simulink model "Feuchtesimulation_G21_EU6AGA_rueckgabewerte"  (R2021b)
settings: Solver=FixedStepAuto  StartTime=start_time  StopTime=stop_time  FixedStep=ts  RelTol=1e-3
undefined symbols (not defined in the file or in its folder): A_Kat0, A_Kat1, A_Kat2, A_Kat3, A_Mantel_Kat0, A_Mantel_Kat1, A_Mantel_Kat2, A_Mantel_Kat3, Air_N2, Air_O2, beladungskennfeld, C_mw, CO2_mw, FeuchteAnsaugluft_rel, FeuchtegradAnsaugluft, Fuel_C, Fuel_H, H2O_mw, H_mw, Kat0_Anzahl_Zonen, Kat1_Anzahl_Zonen, Kat2_Anzahl_Zonen, Kat3_Anzahl_Zonen, l_Kat0, l_Kat1, l_Kat2, l_Kat3, m_Canning_Kat0, m_Canning_Kat1, m_Canning_Kat2, m_Canning_Kat3, m_h2o_kat0_ads, m_h2o_kat0_kond, m_h2o_kat1_ads, m_h2o_kat1_kond, m_h2o_kat2_ads, m_h2o_kat2_kond, m_h2o_kat3_ads, m_h2o_kat3_kond, m_Isolierung_Kat0, m_Isolierung_Kat1, m_Isolierung_Kat2, m_Isolierung_Kat3, m_zeolith_kat0_zone, m_zeolith_kat1_zone, m_zeolith_kat2_zone, m_zeolith_kat3_zone, m_zKat0, m_zKat1, m_zKat2, m_zKat3, Mat_Kat0, Mat_Kat1, Mat_Kat2, Mat_Kat3, N2_mw, O2_mw, p_dsat, Rohr0, Rohr1 ... (+20)
libraries: Feuchtesimulation_Lib x69
(part 2 of 3)

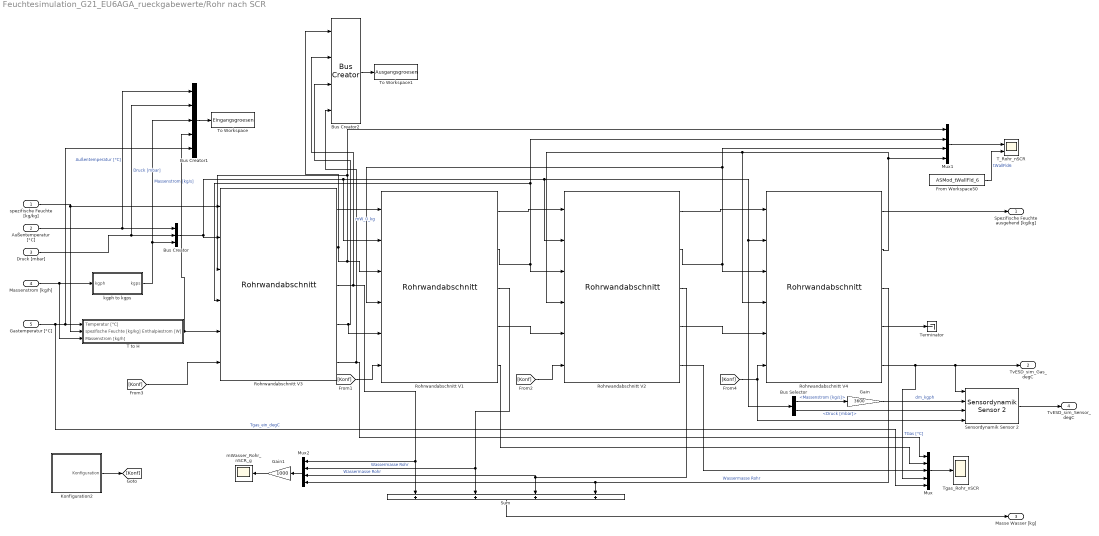
== system Feuchtesimulation_G21_EU6AGA_rueckgabewerte/Rohr nach SCR ==
  spezifische Feuchte [kg/kg] : Inport
  Außentemperatur [°C] : Inport  Port=2
  Druck [mbar] : Inport  Port=3
  Massenstrom [kg/h] : Inport  Port=4
  Gastemperatur [°C] : Inport  Port=5
  Bus Creator : BusCreator  Inputs=3
  Bus Creator1 : BusCreator  Inputs=5
  Bus Creator2 : BusCreator  Inputs=4
  Bus Selector : BusSelector  OutputSignals=Massenstrom [kg/s],Druck [mbar]
  From Workspace50 : FromWorkspace  VariableName=ASMod_tWallFld_6  OutputAfterFinalValue=Holding final value
  Gain : Gain  Gain=3600
  Gain1 : Gain  Gain=1000
  Konfiguration2 : Subsystem
  Mux : Mux  Inputs=5
  Mux1 : Mux
  Mux2 : Mux
  Rohrwandabschnitt V{1..4} (4 alike) : Feuchtesimulation_Lib/Rohrwandabschnitt  SystemSampleTime=-1  VariantActivationTime=update diagram  Latency=0  AutoFrameSizeCalculation=off
  Sensordynamik Sensor 2 : Feuchtesimulation_Lib/Sensordynamik Sensor 2  SystemSampleTime=-1  VariantActivationTime=update diagram  Latency=0  AutoFrameSizeCalculation=off
  Sum : Sum  Inputs=++++
  T to H : Subsystem
  T_Rohr_nSCR : Scope  NumInputPorts=2
  Terminator : Terminator
  Tgas_Rohr_nSCR : Scope
  To Workspace : ToWorkspace  VariableName=Eingangsgroesen  SaveFormat=Structure With Time  SampleTime=-1
  To Workspace1 : ToWorkspace  VariableName=Ausgangsgroesen  SaveFormat=Structure With Time  SampleTime=-1
  kgph to kgps : Subsystem
  mWasser_Rohr_nSCR_g : Scope
  Spezifische Feuchte ausgehend [kg/kg] : Outport  VectorParamsAs1DForOutWhenUnconnected=off
  TvESD_sim_Gas_degC : Outport  Port=2  VectorParamsAs1DForOutWhenUnconnected=off
  Masse Wasser [kg] : Outport  Port=3  VectorParamsAs1DForOutWhenUnconnected=off
  TvESD_sim_Sensor_degC : Outport  Port=4  VectorParamsAs1DForOutWhenUnconnected=off
  wires:
  spezifische Feuchte [kg/kg]/1 -> Rohrwandabschnitt V3/1, T to H/2(spezifische Feuchte [kg/kg])
  Massenstrom [kg/h]/1 -> T to H/3(Massenstrom [kg/h]), kgph to kgps/1(kgph)
  Konfiguration2/1(Konfiguration) -> [Konf]
  Gastemperatur [°C]/1 -> T to H/1(Temperatur [°C]), Bus Creator1/5, Mux/5  "Tgas_ein_degC"
  Rohrwandabschnitt V3/1 -> Rohrwandabschnitt V1/1
  Rohrwandabschnitt V1/1 -> Rohrwandabschnitt V2/1
  Rohrwandabschnitt V2/1 -> Rohrwandabschnitt V4/1
  Rohrwandabschnitt V3/4 -> Bus Creator2/3, Rohrwandabschnitt V1/5
  Rohrwandabschnitt V1/4 -> Rohrwandabschnitt V2/5
  Rohrwandabschnitt V2/4 -> Rohrwandabschnitt V4/5
  [Konf] -> Rohrwandabschnitt V1/6
  [Konf] -> Rohrwandabschnitt V2/6
  [Konf] -> Rohrwandabschnitt V3/6
  Außentemperatur [°C]/1 -> Bus Creator1/1, Bus Creator/1  "Außentemperatur [°C]"
  kgph to kgps/1(kgps) -> Bus Creator/3, Bus Creator1/3  "Massenstrom [kg/s]"
  Druck [mbar]/1 -> Bus Creator/2, Bus Creator1/2  "Druck [mbar]"
  T to H/1(Enthalpiestrom [W]) -> Bus Creator1/4, Rohrwandabschnitt V3/5
  Rohrwandabschnitt V3/2 -> Bus Creator2/1, Mux1/1, Rohrwandabschnitt V3/3, Rohrwandabschnitt V1/3
  Rohrwandabschnitt V1/2 -> Mux1/2, Rohrwandabschnitt V3/4, Rohrwandabschnitt V2/3
  Rohrwandabschnitt V2/2 -> Mux1/3, Rohrwandabschnitt V1/4, Rohrwandabschnitt V4/3
  Rohrwandabschnitt V4/2 -> Mux1/4, Rohrwandabschnitt V4/4, Rohrwandabschnitt V2/4
  Rohrwandabschnitt V4/1 -> Spezifische Feuchte ausgehend [kg/kg]/1
  Rohrwandabschnitt V3/3 -> Bus Creator2/2, Sum/1, Mux2/1  "mW_0_kg"
  Rohrwandabschnitt V1/3 -> Mux2/2, Sum/2  "Wassermasse Rohr"
  Rohrwandabschnitt V2/3 -> Sum/3, Mux2/3  "Wassermasse Rohr"
  Rohrwandabschnitt V4/3 -> Mux2/4, Sum/4  "Wassermasse Rohr"
  Sum/1 -> Masse Wasser [kg]/1
  Rohrwandabschnitt V2/5 -> Mux/3
  Rohrwandabschnitt V3/5 -> Bus Creator2/4, Mux/1
  Rohrwandabschnitt V1/5 -> Mux/2
  Mux/1 -> Tgas_Rohr_nSCR/1
  Rohrwandabschnitt V4/5 -> Mux/4, Sensordynamik Sensor 2/1, TvESD_sim_Gas_degC/1  "TGas [°C]"
  Mux1/1 -> T_Rohr_nSCR/1
  Rohrwandabschnitt V4/4 -> Terminator/1
  From Workspace50/1 -> T_Rohr_nSCR/2  "tWallFld6"
  [Konf] -> Sensordynamik Sensor 2/4, Rohrwandabschnitt V4/6
  Bus Selector/2 -> Sensordynamik Sensor 2/3  "<Druck [mbar]>"
  Bus Selector/1 -> Gain/1  "<Massenstrom [kg/s]>"
  Gain/1 -> Sensordynamik Sensor 2/2  "dm_kgph"
  Sensordynamik Sensor 2/1 -> TvESD_sim_Sensor_degC/1
  Bus Creator/1 -> Rohrwandabschnitt V1/2, Rohrwandabschnitt V2/2, Bus Selector/1, Rohrwandabschnitt V4/2, Rohrwandabschnitt V3/2
  Gain1/1 -> mWasser_Rohr_nSCR_g/1
  Mux2/1 -> Gain1/1
  Bus Creator1/1 -> To Workspace/1
  Bus Creator2/1 -> To Workspace1/1

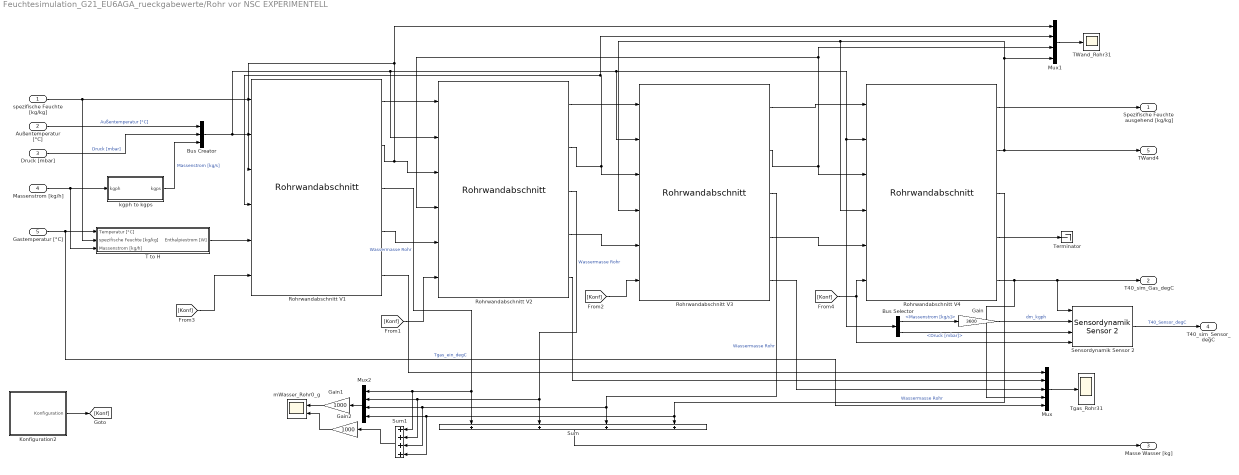
== system Feuchtesimulation_G21_EU6AGA_rueckgabewerte/Rohr vor NSC EXPERIMENTELL ==
  spezifische Feuchte [kg/kg] : Inport
  Außentemperatur [°C] : Inport  Port=2
  Druck [mbar] : Inport  Port=3
  Massenstrom [kg/h] : Inport  Port=4
  Gastemperatur [°C] : Inport  Port=5
  Bus Creator : BusCreator  Inputs=3
  Bus Selector : BusSelector  OutputSignals=Massenstrom [kg/s],Druck [mbar]
  Gain : Gain  Gain=3600
  Gain1 : Gain  Gain=1000
  Gain2 : Gain  Gain=1000
  Konfiguration2 : Subsystem
  Mux : Mux  Inputs=5
  Mux1 : Mux
  Mux2 : Mux
  Rohrwandabschnitt V{1..4} (4 alike) : Feuchtesimulation_Lib/Rohrwandabschnitt  SystemSampleTime=-1  VariantActivationTime=update diagram  Latency=0  AutoFrameSizeCalculation=off
  Sensordynamik Sensor 2 : Feuchtesimulation_Lib/Sensordynamik Sensor 2  SystemSampleTime=-1  VariantActivationTime=update diagram  Latency=0  AutoFrameSizeCalculation=off
  Sum : Sum  Inputs=++++
  Sum1 : Sum  Inputs=4
  T to H : Subsystem
  TWand_Rohr31 : Scope
  Terminator : Terminator
  Tgas_Rohr31 : Scope
  kgph to kgps : Subsystem
  mWasser_Rohr0_g : Scope  NumInputPorts=2
  Spezifische Feuchte ausgehend [kg/kg] : Outport  VectorParamsAs1DForOutWhenUnconnected=off
  T40_sim_Gas_degC : Outport  Port=2  VectorParamsAs1DForOutWhenUnconnected=off
  Masse Wasser [kg] : Outport  Port=3  VectorParamsAs1DForOutWhenUnconnected=off
  T40_sim_Sensor_degC : Outport  Port=4  VectorParamsAs1DForOutWhenUnconnected=off
  TWand4 : Outport  Port=5  VectorParamsAs1DForOutWhenUnconnected=off
  wires:
  spezifische Feuchte [kg/kg]/1 -> Rohrwandabschnitt V1/1, T to H/2(spezifische Feuchte [kg/kg])
  Massenstrom [kg/h]/1 -> T to H/3(Massenstrom [kg/h]), kgph to kgps/1(kgph)
  Konfiguration2/1(Konfiguration) -> [Konf]
  Gastemperatur [°C]/1 -> Mux/5, T to H/1(Temperatur [°C])  "Tgas_ein_degC"
  Rohrwandabschnitt V1/1 -> Rohrwandabschnitt V2/1
  Rohrwandabschnitt V2/1 -> Rohrwandabschnitt V3/1
  Rohrwandabschnitt V3/1 -> Rohrwandabschnitt V4/1
  Rohrwandabschnitt V1/4 -> Rohrwandabschnitt V2/5
  Rohrwandabschnitt V2/4 -> Rohrwandabschnitt V3/5
  Rohrwandabschnitt V3/4 -> Rohrwandabschnitt V4/5
  [Konf] -> Rohrwandabschnitt V2/6
  [Konf] -> Rohrwandabschnitt V3/6
  [Konf] -> Sensordynamik Sensor 2/4, Rohrwandabschnitt V4/6
  [Konf] -> Rohrwandabschnitt V1/6
  Außentemperatur [°C]/1 -> Bus Creator/1  "Außentemperatur [°C]"
  kgph to kgps/1(kgps) -> Bus Creator/3  "Massenstrom [kg/s]"
  Druck [mbar]/1 -> Bus Creator/2  "Druck [mbar]"
  Bus Creator/1 -> Rohrwandabschnitt V2/2, Rohrwandabschnitt V3/2, Bus Selector/1, Rohrwandabschnitt V4/2, Rohrwandabschnitt V1/2
  T to H/1(Enthalpiestrom [W]) -> Rohrwandabschnitt V1/5
  Rohrwandabschnitt V1/2 -> Mux1/1, Rohrwandabschnitt V1/3, Rohrwandabschnitt V2/3
  Rohrwandabschnitt V2/2 -> Mux1/2, Rohrwandabschnitt V1/4, Rohrwandabschnitt V3/3
  Rohrwandabschnitt V3/2 -> Mux1/3, Rohrwandabschnitt V2/4, Rohrwandabschnitt V4/3
  Rohrwandabschnitt V4/2 -> TWand4/1, Mux1/4, Rohrwandabschnitt V4/4, Rohrwandabschnitt V3/4
  Rohrwandabschnitt V4/1 -> Spezifische Feuchte ausgehend [kg/kg]/1
  Rohrwandabschnitt V1/3 -> Sum1/1, Mux2/1, Sum/1  "Wassermasse Rohr"
  Rohrwandabschnitt V2/3 -> Sum/2, Sum1/2, Mux2/2  "Wassermasse Rohr"
  Rohrwandabschnitt V3/3 -> Sum/3, Sum1/3, Mux2/3  "Wassermasse Rohr"
  Rohrwandabschnitt V4/3 -> Sum1/4, Mux2/4, Sum/4  "Wassermasse Rohr"
  Sum/1 -> Masse Wasser [kg]/1
  Rohrwandabschnitt V4/5 -> Mux/4, Sensordynamik Sensor 2/1, T40_sim_Gas_degC/1
  Mux/1 -> Tgas_Rohr31/1
  Rohrwandabschnitt V1/5 -> Mux/1
  Rohrwandabschnitt V2/5 -> Mux/2
  Rohrwandabschnitt V3/5 -> Mux/3
  Mux1/1 -> TWand_Rohr31/1
  Rohrwandabschnitt V4/4 -> Terminator/1
  Bus Selector/1 -> Gain/1  "<Massenstrom [kg/s]>"
  Gain/1 -> Sensordynamik Sensor 2/2  "dm_kgph"
  Bus Selector/2 -> Sensordynamik Sensor 2/3  "<Druck [mbar]>"
  Sensordynamik Sensor 2/1 -> T40_sim_Sensor_degC/1  "T40_Sensor_degC"
  Mux2/1 -> Gain1/1
  Gain1/1 -> mWasser_Rohr0_g/1
  Sum1/1 -> Gain2/1
  Gain2/1 -> mWasser_Rohr0_g/2

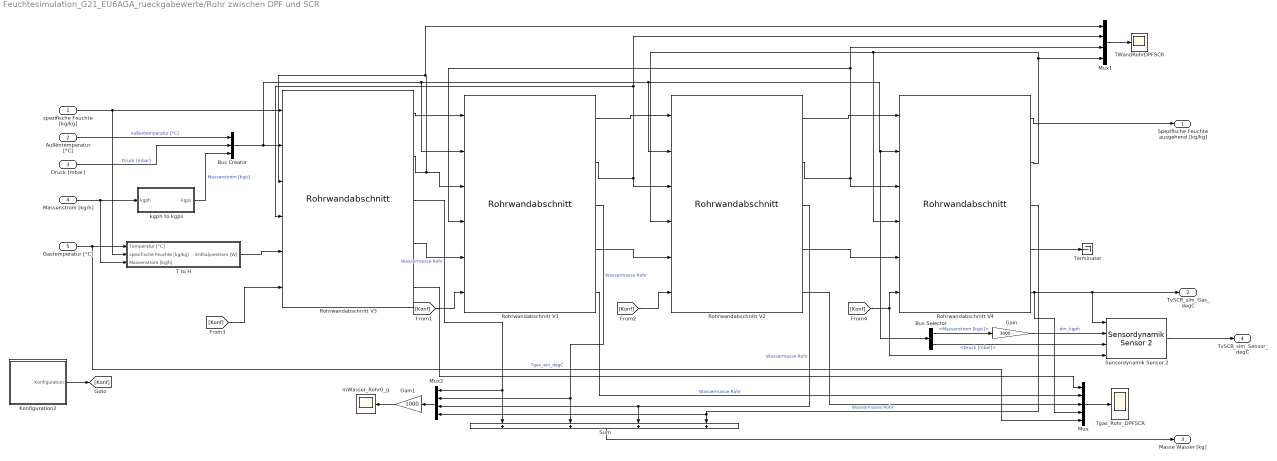
== system Feuchtesimulation_G21_EU6AGA_rueckgabewerte/Rohr zwischen DPF und SCR ==
  spezifische Feuchte [kg/kg] : Inport
  Außentemperatur [°C] : Inport  Port=2
  Druck [mbar] : Inport  Port=3
  Massenstrom [kg/h] : Inport  Port=4
  Gastemperatur [°C] : Inport  Port=5
  Bus Creator : BusCreator  Inputs=3
  Bus Selector : BusSelector  OutputSignals=Massenstrom [kg/s],Druck [mbar]
  Gain : Gain  Gain=3600
  Gain1 : Gain  Gain=1000
  Konfiguration2 : Subsystem
  Mux : Mux  Inputs=5
  Mux1 : Mux
  Mux2 : Mux
  Rohrwandabschnitt V{1..4} (4 alike) : Feuchtesimulation_Lib/Rohrwandabschnitt  SystemSampleTime=-1  VariantActivationTime=update diagram  Latency=0  AutoFrameSizeCalculation=off
  Sensordynamik Sensor 2 : Feuchtesimulation_Lib/Sensordynamik Sensor 2  SystemSampleTime=-1  VariantActivationTime=update diagram  Latency=0  AutoFrameSizeCalculation=off
  Sum : Sum  Inputs=++++
  T to H : Subsystem
  TWandRohrDPFSCR : Scope
  Terminator : Terminator
  Tgas_Rohr_DPFSCR : Scope
  kgph to kgps : Subsystem
  mWasser_Rohr0_g : Scope
  Spezifische Feuchte ausgehend [kg/kg] : Outport  VectorParamsAs1DForOutWhenUnconnected=off
  TvSCR_sim_Gas_degC : Outport  Port=2  VectorParamsAs1DForOutWhenUnconnected=off
  Masse Wasser [kg] : Outport  Port=3  VectorParamsAs1DForOutWhenUnconnected=off
  TvSCR_sim_Sensor_degC : Outport  Port=4  VectorParamsAs1DForOutWhenUnconnected=off
  wires:
  spezifische Feuchte [kg/kg]/1 -> Rohrwandabschnitt V3/1, T to H/2(spezifische Feuchte [kg/kg])
  Massenstrom [kg/h]/1 -> T to H/3(Massenstrom [kg/h]), kgph to kgps/1(kgph)
  Konfiguration2/1(Konfiguration) -> [Konf]
  Gastemperatur [°C]/1 -> Mux/5, T to H/1(Temperatur [°C])  "Tgas_ein_degC"
  Rohrwandabschnitt V3/1 -> Rohrwandabschnitt V1/1
  Rohrwandabschnitt V1/1 -> Rohrwandabschnitt V2/1
  Rohrwandabschnitt V2/1 -> Rohrwandabschnitt V4/1
  Rohrwandabschnitt V3/4 -> Rohrwandabschnitt V1/5
  Rohrwandabschnitt V1/4 -> Rohrwandabschnitt V2/5
  Rohrwandabschnitt V2/4 -> Rohrwandabschnitt V4/5
  [Konf] -> Rohrwandabschnitt V1/6
  [Konf] -> Rohrwandabschnitt V2/6
  [Konf] -> Rohrwandabschnitt V3/6
  Außentemperatur [°C]/1 -> Bus Creator/1  "Außentemperatur [°C]"
  kgph to kgps/1(kgps) -> Bus Creator/3  "Massenstrom [kg/s]"
  Druck [mbar]/1 -> Bus Creator/2  "Druck [mbar]"
  T to H/1(Enthalpiestrom [W]) -> Rohrwandabschnitt V3/5
  Rohrwandabschnitt V3/2 -> Mux1/1, Rohrwandabschnitt V3/3, Rohrwandabschnitt V1/3
  Rohrwandabschnitt V1/2 -> Mux1/2, Rohrwandabschnitt V3/4, Rohrwandabschnitt V2/3
  Rohrwandabschnitt V2/2 -> Mux1/3, Rohrwandabschnitt V1/4, Rohrwandabschnitt V4/3
  Rohrwandabschnitt V4/2 -> Mux1/4, Rohrwandabschnitt V4/4, Rohrwandabschnitt V2/4
  Rohrwandabschnitt V4/1 -> Spezifische Feuchte ausgehend [kg/kg]/1
  Rohrwandabschnitt V2/3 -> Sum/3, Mux2/3  "Wassermasse Rohr"
  Sum/1 -> Masse Wasser [kg]/1
  Mux/1 -> Tgas_Rohr_DPFSCR/1
  Rohrwandabschnitt V3/5 -> Mux/1
  Rohrwandabschnitt V2/5 -> Mux/3
  Rohrwandabschnitt V4/5 -> Sensordynamik Sensor 2/1, TvSCR_sim_Gas_degC/1, Mux/4
  Mux1/1 -> TWandRohrDPFSCR/1
  Rohrwandabschnitt V4/4 -> Terminator/1
  [Konf] -> Sensordynamik Sensor 2/4, Rohrwandabschnitt V4/6
  Bus Selector/2 -> Sensordynamik Sensor 2/3  "<Druck [mbar]>"
  Bus Selector/1 -> Gain/1  "<Massenstrom [kg/s]>"
  Gain/1 -> Sensordynamik Sensor 2/2  "dm_kgph"
  Sensordynamik Sensor 2/1 -> TvSCR_sim_Sensor_degC/1
  Bus Creator/1 -> Rohrwandabschnitt V1/2, Rohrwandabschnitt V2/2, Bus Selector/1, Rohrwandabschnitt V4/2, Rohrwandabschnitt V3/2
  Mux2/1 -> Gain1/1
  Rohrwandabschnitt V4/3 -> Mux2/4, Sum/4  "Wassermasse Rohr"
  Rohrwandabschnitt V3/3 -> Mux2/1, Sum/1  "Wassermasse Rohr"
  Rohrwandabschnitt V1/3 -> Mux2/2, Sum/2  "Wassermasse Rohr"
  Gain1/1 -> mWasser_Rohr0_g/1
  Rohrwandabschnitt V1/5 -> Mux/2  "Wassermasse Rohr"

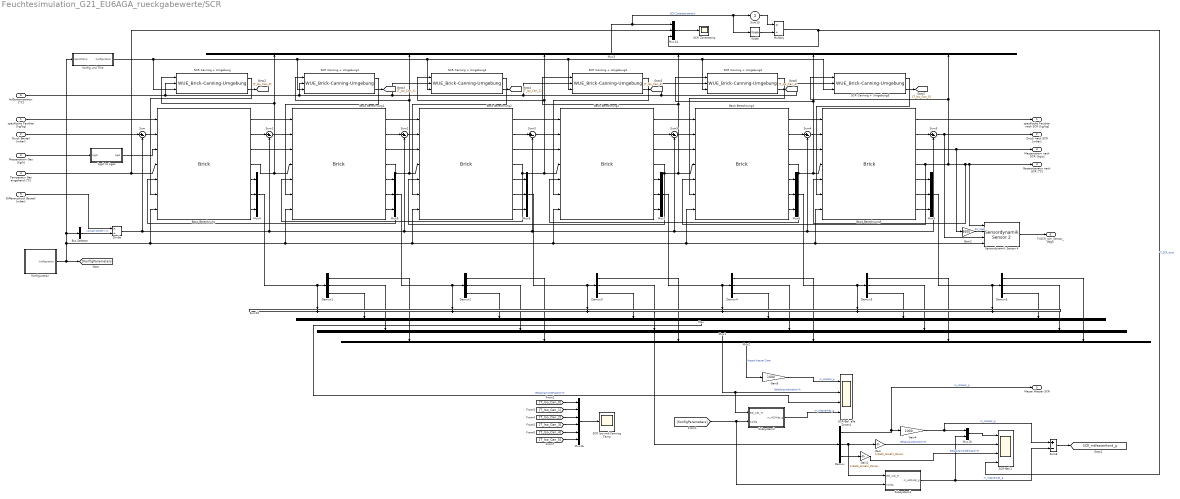
== system Feuchtesimulation_G21_EU6AGA_rueckgabewerte/SCR ==
  spezifische Feuchte [kg/kg] : Inport
  Druck Bauteil [mbar] : Inport  Port=2
  Massenstrom Gas [kg/h] : Inport  Port=3
  Temperatur Gas eingehend [°C] : Inport  Port=4
  Differenzdruck Bauteil [mbar] : Inport  Port=5
  Außentemperatur [°C] : Inport  Port=6
  Basis Berechnung{,1..5} (6 alike) : Feuchtesimulation_Lib/Brick  SystemSampleTime=-1  VariantActivationTime=update diagram  Latency=0  AutoFrameSizeCalculation=off
  Bus Selector : BusSelector  OutputSignals=Anzahl Zonen [-]
  Demux{,1..6} (7 alike) : Demux  Outputs=3
  Divide : Product  Inputs=*/
  Gain : Gain  Gain=1/Kat2_Anzahl_Zonen
  Gain1 : Gain  Gain=1/Kat2_Anzahl_Zonen
  Gain2 : Gain  Gain=3600
  Gain4 : Gain  Gain=1000
  Gain5 : Gain  Gain=1000
  Konfig und TInit : Subsystem
  Konfiguration : Subsystem
  Multiply : Product  Inputs=*/
  Mux{,1..3,16} (5 alike) : Mux  Inputs=6
  Mux10 : Mux  Inputs=2
  Mux{4..9,14} (7 alike) : Mux  Inputs=3
  SCR Canning + Umgebung{,1..5} (6 alike) : Feuchtesimulation_Lib/WUE_Brick-Canning-Umgebung  SystemSampleTime=-1  VariantActivationTime=update diagram  Latency=0  AutoFrameSizeCalculation=off
  SCR Iso-und-CanningTemp : Scope
  SCR Zonentemp : Scope
  SCR-Bel. alle Zonen1 : Scope  NumInputPorts=4
  SCR-Bel.1 : Scope  NumInputPorts=4
  Sensordynamik Sensor 4 : Feuchtesimulation_Lib/Sensordynamik Sensor 2  SystemSampleTime=-1  VariantActivationTime=update diagram  Latency=0  AutoFrameSizeCalculation=off
  Subsystem2 : Subsystem
  Subsystem3 : Subsystem
  Sum{,1..5,9} (7 alike) : Sum  Inputs=|+-
  Sum10 : Sum  Inputs=++++++
  Sum13 : Sum  Inputs=+
  Sum6 : Sum  Inputs=+-
  Width : Width
  kgph to kgps : Subsystem
  spezifische Feuchte nach SCR [kg/kg] : Outport  VectorParamsAs1DForOutWhenUnconnected=off
  Druck nach SCR [mbar] : Outport  Port=2  VectorParamsAs1DForOutWhenUnconnected=off
  Massenstrom nach SCR [kg/s] : Outport  Port=3  VectorParamsAs1DForOutWhenUnconnected=off
  Gastemperatur nach SCR [°C] : Outport  Port=4  VectorParamsAs1DForOutWhenUnconnected=off
  Masse Wasser SCR : Outport  Port=5  VectorParamsAs1DForOutWhenUnconnected=off
  TnSCR_sim_Sensor_degC : Outport  Port=6  VectorParamsAs1DForOutWhenUnconnected=off
  tag scope: SCR_mWasserKond_g=global
  wires:
  Sum10/1 -> Demux/1
  Gain1/1 -> SCR-Bel.1/3  "Beladung Kondensation %"
  Demux/3 -> Gain1/1
  Basis Berechnung3/7 -> Mux7/3
  Basis Berechnung3/5 -> Mux7/1
  Basis Berechnung2/6 -> Mux6/2
  Basis Berechnung4/7 -> Mux8/3
  Basis Berechnung4/5 -> Mux8/1
  Basis Berechnung2/5 -> Mux6/1
  Basis Berechnung4/6 -> Mux8/2
  Basis Berechnung5/5 -> Mux9/1
  Basis Berechnung2/7 -> Mux6/3
  Basis Berechnung1/2 -> Sum2/1
  kgph to kgps/1(kgps) -> Basis Berechnung/3
  Basis Berechnung4/3 -> Basis Berechnung5/3
  Basis Berechnung/5 -> Mux4/1
  Basis Berechnung/6 -> Mux4/2
  Basis Berechnung5/7 -> Mux9/3
  Gain/1 -> SCR-Bel.1/2  "Belatung Adsorption %"
  Basis Berechnung2/1 -> Basis Berechnung3/1
  Massenstrom Gas [kg/h]/1 -> kgph to kgps/1(kgph)
  Sum2/1 -> Basis Berechnung2/2
  Sum1/1 -> Basis Berechnung1/2
  Sum/1 -> Basis Berechnung/2
  Differenzdruck Bauteil [mbar]/1 -> Divide/1
  Basis Berechnung1/7 -> Mux5/3
  Basis Berechnung1/6 -> Mux5/2
  Basis Berechnung1/5 -> Mux5/1
  Basis Berechnung4/1 -> Basis Berechnung5/1
  Basis Berechnung/4 -> Basis Berechnung1/4, SCR Canning + Umgebung/1, Mux3/1
  Basis Berechnung3/6 -> Mux7/2
  Divide/1 -> Sum5/2, Sum4/2, Sum9/2, Sum3/2, Sum2/2, Sum1/2, Sum/2
  Basis Berechnung1/1 -> Basis Berechnung2/1
  Basis Berechnung2/2 -> Sum3/1
  Basis Berechnung3/1 -> Basis Berechnung4/1
  Druck Bauteil [mbar]/1 -> Sum/1
  Basis Berechnung4/2 -> Sum4/1
  Basis Berechnung/1 -> Basis Berechnung1/1
  Basis Berechnung5/2 -> Sum5/1
  Sum4/1 -> Basis Berechnung5/2
  Bus Selector/1 -> Divide/2  "<Anzahl Zonen [-]>"
  Basis Berechnung1/4 -> Basis Berechnung/5, Basis Berechnung2/4, SCR Canning + Umgebung1/1, Mux3/2
  Basis Berechnung2/3 -> Basis Berechnung3/3
  Basis Berechnung2/4 -> Basis Berechnung1/5, Basis Berechnung3/4, Mux3/3, SCR Canning + Umgebung2/1
  Basis Berechnung5/6 -> Mux9/2
  Sum3/1 -> Basis Berechnung3/2
  Basis Berechnung/2 -> Sum1/1
  Basis Berechnung/7 -> Mux4/3
  Basis Berechnung1/3 -> Basis Berechnung2/3
  Basis Berechnung4/4 -> Basis Berechnung3/5, Basis Berechnung5/4, SCR Canning + Umgebung4/1, Mux3/5
  Sum9/1 -> Basis Berechnung4/2
  spezifische Feuchte [kg/kg]/1 -> Basis Berechnung/1
  Basis Berechnung3/4 -> Basis Berechnung4/4, Mux3/4, SCR Canning + Umgebung3/1, Basis Berechnung2/5
  Basis Berechnung3/2 -> Sum9/1
  Basis Berechnung/3 -> Basis Berechnung1/3
  Basis Berechnung5/1 -> spezifische Feuchte nach SCR [kg/kg]/1
  Basis Berechnung3/3 -> Basis Berechnung4/3
  Temperatur Gas eingehend [°C]/1 -> Mux14/2, Basis Berechnung/4
  Demux/1 -> Masse Wasser SCR/1, Gain4/1  "m_Wasser_g"
  Demux1/3 -> Mux/1
  Demux1/2 -> Mux1/1
  Demux1/1 -> Mux2/1
  Demux2/3 -> Mux/2
  Demux2/2 -> Mux1/2
  Demux2/1 -> Mux2/2
  Demux3/3 -> Mux/3
  Demux3/2 -> Mux1/3
  Demux3/1 -> Mux2/3
  Demux4/3 -> Mux/4
  Demux4/2 -> Mux1/4
  Demux4/1 -> Mux2/4
  Demux5/3 -> Mux/5
  Demux5/2 -> Mux1/5
  Demux5/1 -> Mux2/5
  Demux6/3 -> Mux/6
  Demux6/2 -> Mux1/6
  Demux6/1 -> Mux2/6
  Mux2/1 -> Gain5/1  "Masse Wasser Zone"
  Mux1/1 -> SCR-Bel. alle Zonen1/2, Subsystem2/1(Bel_Ads_%)  "Beladung Adsorption %"
  Mux/1 -> SCR-Bel. alle Zonen1/3  "Beladung Kondensation %"
  Außentemperatur [°C]/1 -> SCR Canning + Umgebung5/2, SCR Canning + Umgebung4/2, SCR Canning + Umgebung3/2, SCR Canning + Umgebung2/2, SCR Canning + Umgebung1/2, SCR Canning + Umgebung/2
  SCR Canning + Umgebung/1 -> Basis Berechnung/6
  SCR Canning + Umgebung1/1 -> Basis Berechnung1/6
  SCR Canning + Umgebung2/1 -> Basis Berechnung2/6
  SCR Canning + Umgebung3/1 -> Basis Berechnung3/6
  SCR Canning + Umgebung4/1 -> Basis Berechnung4/6
  SCR Canning + Umgebung5/1 -> Basis Berechnung5/6
  Mux4/1 -> Sum10/1, Demux1/1
  Mux5/1 -> Demux2/1, Sum10/2
  Mux6/1 -> Demux3/1, Sum10/3
  Mux7/1 -> Demux4/1, Sum10/4
  Mux8/1 -> Sum10/5, Demux5/1
  Mux9/1 -> Sum10/6, Demux6/1
  Mux14/1 -> SCR Zonentemp/1
  Demux/2 -> Subsystem3/1(Bel_Ads_%), Gain/1
  Subsystem2/1(m_H2OAds_g) -> SCR-Bel. alle Zonen1/4  "m_WasserAds_g"
  [KonfigParameters] -> Subsystem2/2(Konfig), Subsystem3/2(Konfig)
  Gain5/1 -> SCR-Bel. alle Zonen1/1  "m_Wasser_g"
  Mux10/1 -> SCR-Bel.1/1
  Subsystem3/1(m_H2OAds_g) -> Sum6/2, Mux10/2  "m_WasserAds_g"
  Sum6/1 -> [SCR_mWasserKond_g]
  Gain4/1 -> Sum6/1, Mux10/1  "m_Wasser_g"
  Sum13/1 -> Multiply/1
  Width/1 -> Multiply/2
  Multiply/1 -> SCR-Bel.1/4, Mux14/3  "T_SCR_avrg"
  Mux3/1 -> Sum13/1, Width/1, Mux14/1  "SCR Zonentemperatur"
  Konfig und TInit/1(Konfiguration) -> SCR Canning + Umgebung2/3, SCR Canning + Umgebung3/3, SCR Canning + Umgebung4/3, SCR Canning + Umgebung5/3, SCR Canning + Umgebung1/3, SCR Canning + Umgebung/3
  [T_Iso_Can_3] -> Mux16/4
  [T_Iso_Can_2] -> Mux16/3
  [T_Iso_Can_0] -> Mux16/1
  [T_Iso_Can_5] -> Mux16/6
  [T_Iso_Can_4] -> Mux16/5
  [T_Iso_Can_1] -> Mux16/2
  Mux16/1 -> SCR Iso-und-CanningTemp/1
  SCR Canning + Umgebung/2 -> [T_Iso_Can_0]
  SCR Canning + Umgebung1/2 -> [T_Iso_Can_1]
  SCR Canning + Umgebung2/2 -> [T_Iso_Can_2]
  SCR Canning + Umgebung3/2 -> [T_Iso_Can_3]
  SCR Canning + Umgebung4/2 -> [T_Iso_Can_4]
  SCR Canning + Umgebung5/2 -> [T_Iso_Can_5]
  Sum5/1 -> Sensordynamik Sensor 4/3, Druck nach SCR [mbar]/1
  Basis Berechnung5/3 -> Gain2/1, Massenstrom nach SCR [kg/s]/1
  Gain2/1 -> Sensordynamik Sensor 4/2  "dm_kgph"
  Sensordynamik Sensor 4/1 -> TnSCR_sim_Sensor_degC/1
  Basis Berechnung5/4 -> Basis Berechnung4/5, SCR Canning + Umgebung5/1, Mux3/6, Basis Berechnung5/5, Sensordynamik Sensor 4/1, Gastemperatur nach SCR [°C]/1
  Konfiguration/1(Konfiguration) -> [KonfigParameters], Basis Berechnung/7, Sensordynamik Sensor 4/4, Basis Berechnung5/7, Basis Berechnung4/7, Basis Berechnung3/7, Basis Berechnung2/7, Basis Berechnung1/7, Konfig und TInit/1(ReInitTemp), Bus Selector/1

== system Feuchtesimulation_G21_EU6AGA_rueckgabewerte/Subsystem ==
  spez-Feuchte [kg/kg] : Inport
  spez-Feuchte Verbrennung only [kg/kg] : Inport  Port=2
  mf_Abgas [kg/h] : Inport  Port=3
  Gain : Gain  Gain=1000
  Gain1 : Gain  Gain=1000
  Gain2 : Gain  Gain=1/3600
  Gain3 : Gain  Gain=1/3600
  Integrator : Integrator
  Integrator1 : Integrator
  Multiply : Product
  Multiply1 : Product
  mH2O [g] : Outport  VectorParamsAs1DForOutWhenUnconnected=off
  mH2O Verbr.-only [g] : Outport  Port=2  VectorParamsAs1DForOutWhenUnconnected=off
  wires:
  Multiply/1 -> Gain/1
  spez-Feuchte [kg/kg]/1 -> Multiply/1
  spez-Feuchte Verbrennung only [kg/kg]/1 -> Multiply1/2
  mf_Abgas [kg/h]/1 -> Multiply/2, Multiply1/1
  Gain/1 -> Gain2/1  "Wassermassenstrom_gesamt [g/h]"
  Multiply1/1 -> Gain1/1
  Gain1/1 -> Gain3/1  "Wassermassenstrom_Verbrennung-only [g/h]"
  Integrator/1 -> mH2O [g]/1
  Integrator1/1 -> mH2O Verbr.-only [g]/1
  Gain2/1 -> Integrator/1
  Gain3/1 -> Integrator1/1

== system Feuchtesimulation_G21_EU6AGA_rueckgabewerte/TempResetTrigger ==
  Constant : Constant  Value=45
  Constant1 : Constant  Value=3
  Data Type Conversion : DataTypeConversion  OutDataTypeStr=double
  From Workspace : FromWorkspace  VariableName=CoEng_st  Interpolate=off  OutputAfterFinalValue=Holding final value
  From Workspace1 : FromWorkspace  VariableName=EngDa_tEng  Interpolate=off  OutputAfterFinalValue=Holding final value
  Logical Operator : Logic  AllPortsSameDT=off  OutDataTypeStr=boolean
  Relational Operator : RelationalOperator  Operator=<  OutDataTypeStr=boolean  RndMeth=Simplest
  Relational Operator1 : RelationalOperator  Operator=<  OutDataTypeStr=boolean  RndMeth=Simplest
  Scope : Scope  NumInputPorts=2
  Resi : Outport  VectorParamsAs1DForOutWhenUnconnected=off
  wires:
  From Workspace/1 -> Relational Operator/1  "CoEng_st"
  Constant1/1 -> Relational Operator/2
  Constant/1 -> Relational Operator1/2
  From Workspace1/1 -> Scope/2, Relational Operator1/1
  Relational Operator/1 -> Logical Operator/1
  Relational Operator1/1 -> Logical Operator/2
  Logical Operator/1 -> Data Type Conversion/1
  Data Type Conversion/1 -> Scope/1, Resi/1

== system Feuchtesimulation_G21_EU6AGA_rueckgabewerte/ASC/Konfig und TInit ==
  ReInitTemp : Inport
  Bus Creator : BusCreator  Inputs=7
  Bus Selector : BusSelector  OutputSignals=Re-InitialisierungsTemp [degC]
  Constant : Constant  Value=RTh_Brick_Iso_Kat3
  Constant1 : Constant  Value=RTh_Iso_Canning_Kat3
  Constant2 : Constant  Value=m_Isolierung_Kat3
  Constant3 : Constant  Value=m_Canning_Kat3
  Constant4 : Constant  Value=A_Mantel_Kat3
  Constant5 : Constant  Value=Kat3_Anzahl_Zonen
  Konfiguration : Outport  VectorParamsAs1DForOutWhenUnconnected=off
  wires:
  Bus Creator/1 -> Konfiguration/1
  Constant/1 -> Bus Creator/1  "RTh_Brick_Iso [K/W]"
  Constant1/1 -> Bus Creator/2  "RTh_Iso_Canning [K/W]"
  Constant3/1 -> Bus Creator/4  "m_Canning [kg]"
  Constant4/1 -> Bus Creator/5  "A_Mantel [m2]"
  Constant5/1 -> Bus Creator/6  "Anzahl_Zonen [-]"
  Constant2/1 -> Bus Creator/3  "m_Isolierung [kg]"
  ReInitTemp/1 -> Bus Selector/1
  Bus Selector/1 -> Bus Creator/7  "<Re-InitialisierungsTemp [degC]>"

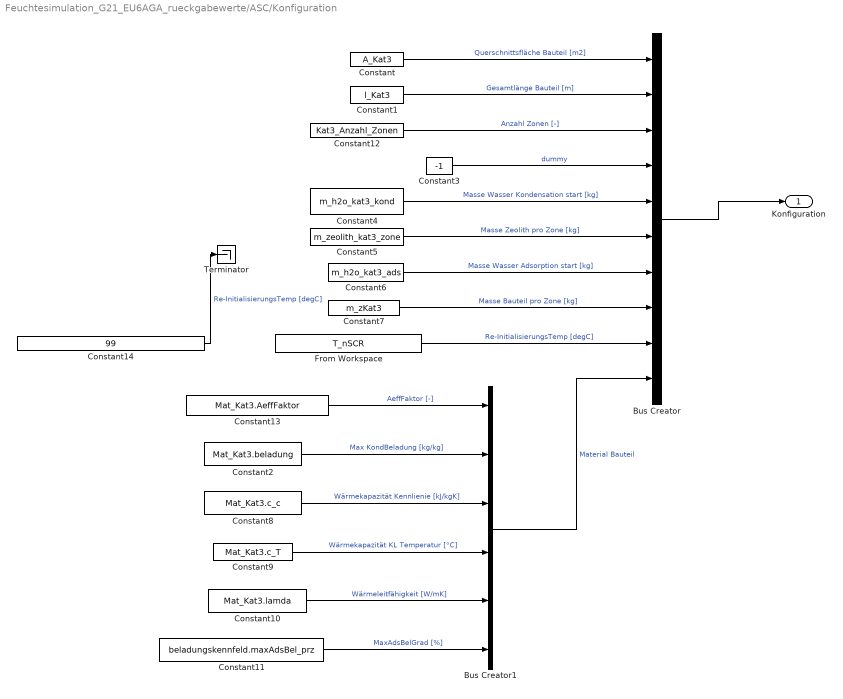
== system Feuchtesimulation_G21_EU6AGA_rueckgabewerte/ASC/Konfiguration ==
  Bus Creator : BusCreator  Inputs=10
  Bus Creator1 : BusCreator  Inputs=6
  Constant : Constant  Value=A_Kat3
  Constant1 : Constant  Value=l_Kat3
  Constant10 : Constant  Value=Mat_Kat3.lamda
  Constant11 : Constant  Value=beladungskennfeld.maxAdsBel_prz
  Constant12 : Constant  Value=Kat3_Anzahl_Zonen
  Constant13 : Constant  Value=Mat_Kat3.AeffFaktor
  Constant14 : Constant  Value=99
  Constant2 : Constant  Value=Mat_Kat3.beladung
  Constant3 : Constant  Value=-1
  Constant4 : Constant  Value=m_h2o_kat3_kond
  Constant5 : Constant  Value=m_zeolith_kat3_zone
  Constant6 : Constant  Value=m_h2o_kat3_ads
  Constant7 : Constant  Value=m_zKat3
  Constant8 : Constant  Value=Mat_Kat3.c_c
  Constant9 : Constant  Value=Mat_Kat3.c_T
  From Workspace : FromWorkspace  VariableName=T_nSCR
  Terminator : Terminator
  Konfiguration : Outport  VectorParamsAs1DForOutWhenUnconnected=off
  wires:
  Constant10/1 -> Bus Creator1/5  "Wärmeleitfähigkeit [W/mK]"
  Constant7/1 -> Bus Creator/8  "Masse Bauteil pro Zone [kg]"
  Bus Creator1/1 -> Bus Creator/10  "Material Bauteil"
  Constant1/1 -> Bus Creator/2  "Gesamtlänge Bauteil [m]"
  Constant12/1 -> Bus Creator/3  "Anzahl Zonen [-]"
  Bus Creator/1 -> Konfiguration/1
  Constant9/1 -> Bus Creator1/4  "Wärmekapazität KL Temperatur [°C]"
  Constant8/1 -> Bus Creator1/3  "Wärmekapazität Kennlienie [kJ/kgK]"
  Constant2/1 -> Bus Creator1/2  "Max KondBeladung [kg/kg]"
  Constant5/1 -> Bus Creator/6  "Masse Zeolith pro Zone [kg]"
  Constant4/1 -> Bus Creator/5  "Masse Wasser Kondensation start [kg]"
  Constant6/1 -> Bus Creator/7  "Masse Wasser Adsorption start [kg]"
  Constant/1 -> Bus Creator/1  "Querschnittsfläche Bauteil [m2]"
  Constant13/1 -> Bus Creator1/1  "AeffFaktor [-]"
  Constant11/1 -> Bus Creator1/6  "MaxAdsBelGrad [%]"
  From Workspace/1 -> Bus Creator/9  "Re-InitialisierungsTemp [degC]"
  Constant3/1 -> Bus Creator/4  "dummy"
  Constant14/1 -> Terminator/1  "Re-InitialisierungsTemp [degC]"

== system Feuchtesimulation_G21_EU6AGA_rueckgabewerte/ASC/Subsystem2 ==
  Bel_Ads_% : Inport
  Konfig : Inport  Port=2
  Bus Selector : BusSelector  OutputSignals=Masse Zeolith pro Zone [kg],Material Bauteil.MaxAdsBelGrad [%]
  Gain4 : Gain  Gain=0.1
  Multiply : Product  Inputs=3
  m_H2OAds_g : Outport  VectorParamsAs1DForOutWhenUnconnected=off
  wires:
  Gain4/1 -> m_H2OAds_g/1  "m_Wasser_g"
  Konfig/1 -> Bus Selector/1
  Bel_Ads_%/1 -> Multiply/1
  Bus Selector/2 -> Multiply/3  "<MaxAdsBelGrad [%]>"
  Bus Selector/1 -> Multiply/2  "<Masse Zeolith pro Zone [kg]>"
  Multiply/1 -> Gain4/1  "m*10000_kg"

== system Feuchtesimulation_G21_EU6AGA_rueckgabewerte/ASC/Subsystem3 ==
  Bel_Ads_% : Inport
  Konfig : Inport  Port=2
  Bus Selector : BusSelector  OutputSignals=Masse Zeolith pro Zone [kg],Material Bauteil.MaxAdsBelGrad [%]
  Gain4 : Gain  Gain=0.1
  Multiply : Product  Inputs=3
  m_H2OAds_g : Outport  VectorParamsAs1DForOutWhenUnconnected=off
  wires:
  Gain4/1 -> m_H2OAds_g/1  "m_Wasser_g"
  Konfig/1 -> Bus Selector/1
  Bel_Ads_%/1 -> Multiply/1
  Bus Selector/2 -> Multiply/3  "<MaxAdsBelGrad [%]>"
  Bus Selector/1 -> Multiply/2  "<Masse Zeolith pro Zone [kg]>"
  Multiply/1 -> Gain4/1  "m*10000_kg"

== system Feuchtesimulation_G21_EU6AGA_rueckgabewerte/ASC/kgph to kgps ==
  kgph : Inport
  Constant : Constant  Value=3600
  dm_kgps : Product  Inputs=*/
  kgps : Outport  VectorParamsAs1DForOutWhenUnconnected=off
  wires:
  Constant/1 -> dm_kgps/2
  kgph/1 -> dm_kgps/1
  dm_kgps/1 -> kgps/1

== system Feuchtesimulation_G21_EU6AGA_rueckgabewerte/DPF/Konfig und TInit ==
  ReInitTemp : Inport
  Bus Creator : BusCreator  Inputs=7
  Bus Selector : BusSelector  OutputSignals=Re-InitialisierungsTemp [degC]
  Constant : Constant  Value=RTh_Brick_Iso_Kat1
  Constant1 : Constant  Value=RTh_Iso_Canning_Kat1
  Constant2 : Constant  Value=m_Isolierung_Kat1
  Constant3 : Constant  Value=m_Canning_Kat1
  Constant4 : Constant  Value=A_Mantel_Kat1
  Constant5 : Constant  Value=Kat1_Anzahl_Zonen
  Konfiguration : Outport  VectorParamsAs1DForOutWhenUnconnected=off
  wires:
  Bus Creator/1 -> Konfiguration/1
  Constant/1 -> Bus Creator/1  "RTh_Brick_Iso [K/W]"
  Constant1/1 -> Bus Creator/2  "RTh_Iso_Canning [K/W]"
  Constant3/1 -> Bus Creator/4  "m_Canning [kg]"
  Constant4/1 -> Bus Creator/5  "A_Mantel [m2]"
  Constant5/1 -> Bus Creator/6  "Anzahl_Zonen [-]"
  Constant2/1 -> Bus Creator/3  "m_Isolierung [kg]"
  ReInitTemp/1 -> Bus Selector/1
  Bus Selector/1 -> Bus Creator/7  "<Re-InitialisierungsTemp [degC]>"

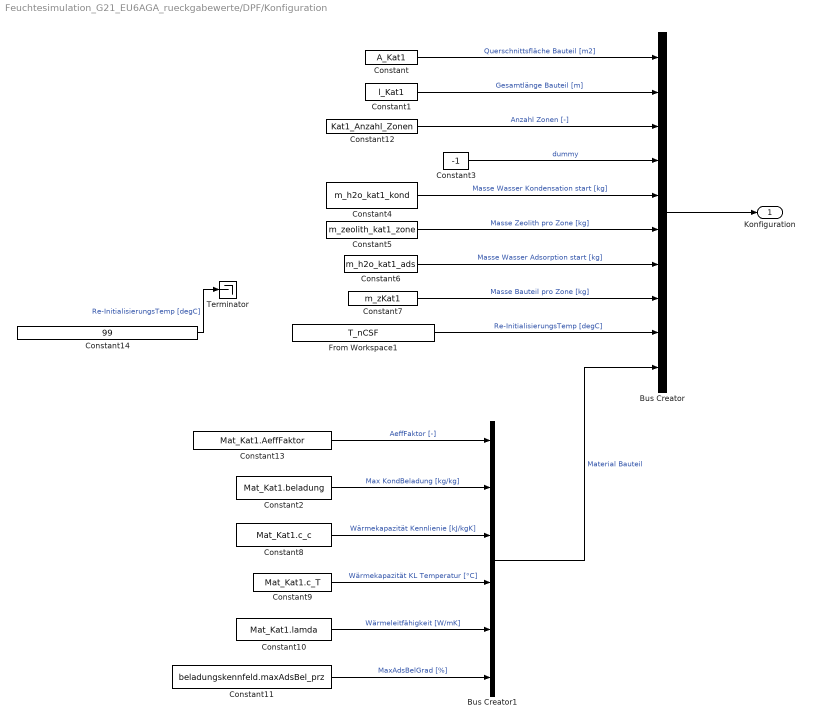
== system Feuchtesimulation_G21_EU6AGA_rueckgabewerte/DPF/Konfiguration ==
  Bus Creator : BusCreator  Inputs=10
  Bus Creator1 : BusCreator  Inputs=6
  Constant : Constant  Value=A_Kat1
  Constant1 : Constant  Value=l_Kat1
  Constant10 : Constant  Value=Mat_Kat1.lamda
  Constant11 : Constant  Value=beladungskennfeld.maxAdsBel_prz
  Constant12 : Constant  Value=Kat1_Anzahl_Zonen
  Constant13 : Constant  Value=Mat_Kat1.AeffFaktor
  Constant14 : Constant  Value=99
  Constant2 : Constant  Value=Mat_Kat1.beladung
  Constant3 : Constant  Value=-1
  Constant4 : Constant  Value=m_h2o_kat1_kond
  Constant5 : Constant  Value=m_zeolith_kat1_zone
  Constant6 : Constant  Value=m_h2o_kat1_ads
  Constant7 : Constant  Value=m_zKat1
  Constant8 : Constant  Value=Mat_Kat1.c_c
  Constant9 : Constant  Value=Mat_Kat1.c_T
  From Workspace1 : FromWorkspace  VariableName=T_nCSF
  Terminator : Terminator
  Konfiguration : Outport  VectorParamsAs1DForOutWhenUnconnected=off
  wires:
  Constant10/1 -> Bus Creator1/5  "Wärmeleitfähigkeit [W/mK]"
  Constant7/1 -> Bus Creator/8  "Masse Bauteil pro Zone [kg]"
  Bus Creator1/1 -> Bus Creator/10  "Material Bauteil"
  Constant1/1 -> Bus Creator/2  "Gesamtlänge Bauteil [m]"
  Constant12/1 -> Bus Creator/3  "Anzahl Zonen [-]"
  Bus Creator/1 -> Konfiguration/1
  Constant9/1 -> Bus Creator1/4  "Wärmekapazität KL Temperatur [°C]"
  Constant8/1 -> Bus Creator1/3  "Wärmekapazität Kennlienie [kJ/kgK]"
  Constant5/1 -> Bus Creator/6  "Masse Zeolith pro Zone [kg]"
  Constant4/1 -> Bus Creator/5  "Masse Wasser Kondensation start [kg]"
  Constant6/1 -> Bus Creator/7  "Masse Wasser Adsorption start [kg]"
  Constant/1 -> Bus Creator/1  "Querschnittsfläche Bauteil [m2]"
  Constant13/1 -> Bus Creator1/1  "AeffFaktor [-]"
  Constant2/1 -> Bus Creator1/2  "Max KondBeladung [kg/kg]"
  Constant11/1 -> Bus Creator1/6  "MaxAdsBelGrad [%]"
  From Workspace1/1 -> Bus Creator/9  "Re-InitialisierungsTemp [degC]"
  Constant3/1 -> Bus Creator/4  "dummy"
  Constant14/1 -> Terminator/1  "Re-InitialisierungsTemp [degC]"

== system Feuchtesimulation_G21_EU6AGA_rueckgabewerte/DPF/Subsystem ==
  Bel_Ads_% : Inport
  Konfig : Inport  Port=2
  Bus Selector : BusSelector  OutputSignals=Masse Zeolith pro Zone [kg],Material Bauteil.MaxAdsBelGrad [%]
  Gain4 : Gain  Gain=0.1
  Multiply : Product  Inputs=3
  m_H2OAds_g : Outport  VectorParamsAs1DForOutWhenUnconnected=off
  wires:
  Gain4/1 -> m_H2OAds_g/1  "m_Wasser_g"
  Konfig/1 -> Bus Selector/1
  Bel_Ads_%/1 -> Multiply/1
  Bus Selector/2 -> Multiply/3  "<MaxAdsBelGrad [%]>"
  Bus Selector/1 -> Multiply/2  "<Masse Zeolith pro Zone [kg]>"
  Multiply/1 -> Gain4/1  "m*10000_kg"

== system Feuchtesimulation_G21_EU6AGA_rueckgabewerte/DPF/Subsystem1 ==
  Bel_Ads_% : Inport
  Konfig : Inport  Port=2
  Bus Selector : BusSelector  OutputSignals=Masse Zeolith pro Zone [kg],Material Bauteil.MaxAdsBelGrad [%]
  Gain4 : Gain  Gain=0.1
  Multiply : Product  Inputs=3
  m_H2OAds_g : Outport  VectorParamsAs1DForOutWhenUnconnected=off
  wires:
  Gain4/1 -> m_H2OAds_g/1  "m_Wasser_g"
  Konfig/1 -> Bus Selector/1
  Bel_Ads_%/1 -> Multiply/1
  Bus Selector/2 -> Multiply/3  "<MaxAdsBelGrad [%]>"
  Bus Selector/1 -> Multiply/2  "<Masse Zeolith pro Zone [kg]>"
  Multiply/1 -> Gain4/1  "m*10000_kg"

== system Feuchtesimulation_G21_EU6AGA_rueckgabewerte/DPF/kgph to kgps ==
  kgph : Inport
  Constant : Constant  Value=3600
  dm_kgps : Product  Inputs=*/
  kgps : Outport  VectorParamsAs1DForOutWhenUnconnected=off
  wires:
  Constant/1 -> dm_kgps/2
  kgph/1 -> dm_kgps/1
  dm_kgps/1 -> kgps/1

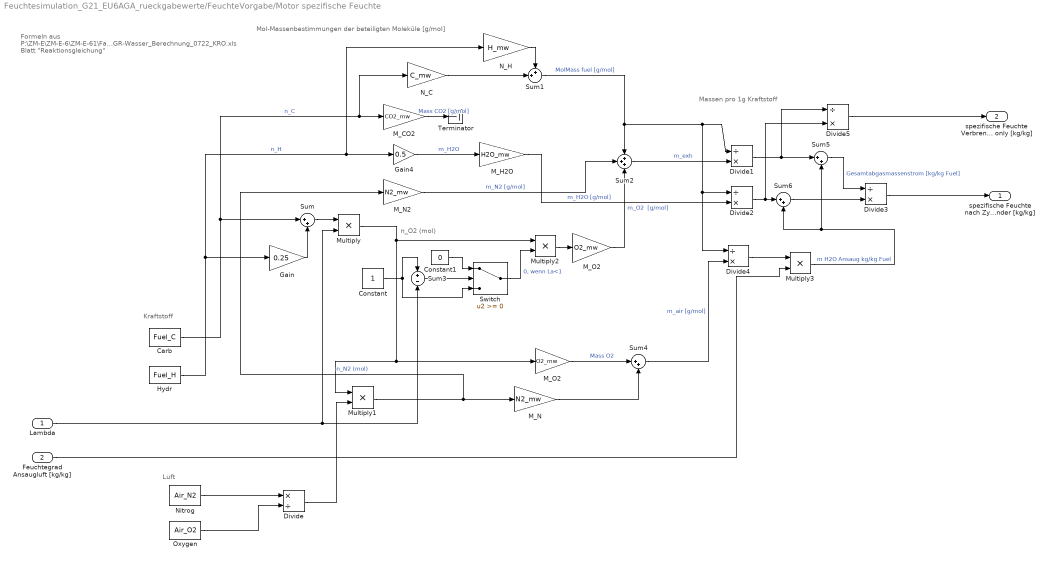
== system Feuchtesimulation_G21_EU6AGA_rueckgabewerte/FeuchteVorgabe/Motor spezifische Feuchte ==
  note: Formeln aus
      | P:\ZM-E\ZM-E-6\ZM-E-61\Fachthemen\Berechnungen\2019_Kondensation-NDAGR-Wasser_Berechnung_0722_KRO.xls
      | Blatt "Reaktionsgleichung"
  note: n_O2 (mol)
  note: Kraftstoff
  note: Luft
  note: Mol-Massenbestimmungen der beteiligten Moleküle [g/mol]
  note: Massen pro 1g Kraftstoff
  Lambda : Inport
  Feuchtegrad Ansaugluft [kg/kg] : Inport  Port=2
  Carb : Constant  Value=Fuel_C
  Constant : Constant
  Constant1 : Constant  Value=0
  Divide : Product  Inputs=*/
  Divide{1..5} (5 alike) : Product  Inputs=/*
  Gain : Gain  Gain=0.25
  Gain4 : Gain  Gain=0.5
  Hydr : Constant  Value=Fuel_H
  M_CO2 : Gain  Gain=CO2_mw
  M_H2O : Gain  Gain=H2O_mw
  M_N : Gain  Gain=N2_mw
  M_N2 : Gain  Gain=N2_mw
  M_O2 : Gain  Gain=O2_mw
  "M_O2 " : Gain  Gain=O2_mw
  Multiply{,1..3} (4 alike) : Product
  N_C : Gain  Gain=C_mw
  N_H : Gain  Gain=H_mw
  Nitrog : Constant  Value=Air_N2
  Oxygen : Constant  Value=Air_O2
  Sum{,4..6} (4 alike) : Sum  Inputs=|++
  Sum1 : Sum  Inputs=++|
  Sum2 : Sum  Inputs=+++
  Sum3 : Sum  Inputs=+-
  Switch : Switch
  Terminator : Terminator
  spezifische Feuchte nach Zylinder [kg/kg] : Outport  VectorParamsAs1DForOutWhenUnconnected=off
  spezifische Feuchte Verbrennung only [kg/kg] : Outport  Port=2  VectorParamsAs1DForOutWhenUnconnected=off
  wires:
  Divide3/1 -> spezifische Feuchte nach Zylinder [kg/kg]/1
  Divide4/1 -> Multiply3/1
  Constant1/1 -> Switch/1
  Sum5/1 -> Divide3/1  "Gesamtabgasmassenstrom [kg/kg Fuel]"
  M_N/1 -> Sum4/2
  "M_O2 "/1 -> Sum4/1  "Mass O2"
  N_C/1 -> Sum1/2
  N_H/1 -> Sum1/1
  Divide2/1 -> Divide5/2, Sum6/1
  Feuchtegrad Ansaugluft [kg/kg]/1 -> Multiply3/2
  Sum4/1 -> Divide4/2  "m_air [g/mol]"
  Sum1/1 -> Sum2/1, Divide4/1, Divide2/1, Divide1/1  "MolMass fuel [g/mol]"
  Sum2/1 -> Divide1/2  "m_exh"
  M_O2/1 -> Sum2/3  "m_O2  [g/mol]"
  Multiply2/1 -> M_O2/1
  Sum3/1 -> Switch/2
  Constant/1 -> Switch/3, Sum3/1
  M_N2/1 -> Sum2/2  "m_N2 [g/mol]"
  M_H2O/1 -> Divide2/2  "m_H2O [g/mol]"
  Multiply1/1 -> M_N/1, M_N2/1  "n_N2 (mol)"
  Divide/1 -> Multiply1/2
  Multiply/1 -> Multiply2/1, Multiply1/1, "M_O2 "/1
  Oxygen/1 -> Divide/2
  Nitrog/1 -> Divide/1
  Sum/1 -> Multiply/1
  Gain/1 -> Sum/2
  Carb/1 -> N_C/1, M_CO2/1, Sum/1  "n_C"
  Hydr/1 -> N_H/1, Gain4/1, Gain/1  "n_H"
  Gain4/1 -> M_H2O/1  "m_H2O"
  Switch/1 -> Multiply2/2  "0, wenn La<1"
  Lambda/1 -> Sum3/2, Multiply/2
  Multiply3/1 -> Sum6/2, Sum5/2  "m H2O Ansaug kg/kg Fuel"
  Sum6/1 -> Divide3/2
  Divide1/1 -> Divide5/1, Sum5/1
  Divide5/1 -> spezifische Feuchte Verbrennung only [kg/kg]/1
  M_CO2/1 -> Terminator/1  "Mass CO2 [g/mol]"

== system Feuchtesimulation_G21_EU6AGA_rueckgabewerte/FeuchteVorgabe/Subsystem ==
  Umgebungsdruck [mbar] : Inport
  Temperatur Ansaugluft [°C] : Inport  Port=2
  relative Luftfeuchte Ansaugluft [-] : Inport  Port=3
  Mischverhältnis Ansaugluft : MATLAB Function  TreatAsAtomicUnit=on
  pdsat : Lookup_n-D  NumberOfTableDimensions=1  BreakpointsForDimension1=p_dsat.T  Table=p_dsat.p  InternalRulePriority=Speed  RndMeth=Simplest  InputSameDT=on
  Feuchtegrad Ansaugluft [kg/kg] : Outport  VectorParamsAs1DForOutWhenUnconnected=off
  wires:
  Temperatur Ansaugluft [°C]/1 -> pdsat/1
  relative Luftfeuchte Ansaugluft [-]/1 -> Mischverhältnis Ansaugluft/1(phi)
  Mischverhältnis Ansaugluft/1(x) -> Feuchtegrad Ansaugluft [kg/kg]/1
  Umgebungsdruck [mbar]/1 -> Mischverhältnis Ansaugluft/3(p_0)
  pdsat/1 -> Mischverhältnis Ansaugluft/2(p_dsat)

== system Feuchtesimulation_G21_EU6AGA_rueckgabewerte/FeuchteVorgabe/Subsystem1 ==
  >=0.1 : Saturate  UpperLimit=9999  LowerLimit=0.1
  >=1 : Saturate  UpperLimit=9999  LowerLimit=1
  Constant : Constant  Value=14.5
  Divide : Product  Inputs=*/
  Divide1 : Product  Inputs=*/
  From Workspace1 : FromWorkspace  VariableName=InjCtl_qSetUnBal
  From Workspace2 : FromWorkspace  VariableName=AFS_dm
  From Workspace3 : FromWorkspace  VariableName=Epm_nEng
  Gain : Gain  Gain=100000/12
  Multiply : Product
  Scope : Scope  NumInputPorts=2
  nantozero1 : Subsystem  AncestorBlock=Kats/Kat2/Wassermenge/nantozero1
  Lambda : Outport  VectorParamsAs1DForOutWhenUnconnected=off
  wires:
  From Workspace1/1 -> Multiply/1  "mg"
  Constant/1 -> Multiply/2
  Divide/1 -> Lambda/1
  nantozero1/1(output) -> Divide/1
  From Workspace2/1 -> Divide1/1, Scope/1  "kg/h"
  Divide1/1 -> Gain/1
  Gain/1 -> nantozero1/1(input)
  From Workspace3/1 -> >=1/1, Scope/2  "rpm"
  >=1/1 -> Divide1/2
  Multiply/1 -> >=0.1/1
  >=0.1/1 -> Divide/2

== system Feuchtesimulation_G21_EU6AGA_rueckgabewerte/FeuchteVorgabe/Subsystem2 ==
  Umgebungsdruck [mbar] : Inport
  Temperatur Ansaugluft [°C] : Inport  Port=2
  relative Luftfeuchte Ansaugluft [-] : Inport  Port=3
  Mischverhältnis Ansaugluft : MATLAB Function  TreatAsAtomicUnit=on
  pdsat : Lookup_n-D  NumberOfTableDimensions=1  BreakpointsForDimension1=p_dsat.T  Table=p_dsat.p  InternalRulePriority=Speed  RndMeth=Simplest  InputSameDT=on
  Feuchtegrad Ansaugluft [kg/kg] : Outport  VectorParamsAs1DForOutWhenUnconnected=off
  wires:
  Temperatur Ansaugluft [°C]/1 -> pdsat/1
  relative Luftfeuchte Ansaugluft [-]/1 -> Mischverhältnis Ansaugluft/1(phi)
  Mischverhältnis Ansaugluft/1(x) -> Feuchtegrad Ansaugluft [kg/kg]/1
  Umgebungsdruck [mbar]/1 -> Mischverhältnis Ansaugluft/3(p_0)
  pdsat/1 -> Mischverhältnis Ansaugluft/2(p_dsat)

== system Feuchtesimulation_G21_EU6AGA_rueckgabewerte/NSC/Konfig und TInit ==
  ReInitTemp : Inport
  Bus Creator : BusCreator  Inputs=7
  Bus Selector : BusSelector  OutputSignals=Re-InitialisierungsTemp [degC]
  Constant : Constant  Value=RTh_Brick_Iso_Kat0
  Constant1 : Constant  Value=RTh_Iso_Canning_Kat0
  Constant2 : Constant  Value=m_Isolierung_Kat0
  Constant3 : Constant  Value=m_Canning_Kat0
  Constant4 : Constant  Value=A_Mantel_Kat0
  Constant5 : Constant  Value=Kat0_Anzahl_Zonen
  Konfiguration : Outport  VectorParamsAs1DForOutWhenUnconnected=off
  wires:
  Bus Creator/1 -> Konfiguration/1
  Constant/1 -> Bus Creator/1  "RTh_Brick_Iso [K/W]"
  Constant1/1 -> Bus Creator/2  "RTh_Iso_Canning [K/W]"
  Constant3/1 -> Bus Creator/4  "m_Canning [kg]"
  Constant4/1 -> Bus Creator/5  "A_Mantel [m2]"
  Constant5/1 -> Bus Creator/6  "Anzahl_Zonen [-]"
  Constant2/1 -> Bus Creator/3  "m_Isolierung [kg]"
  ReInitTemp/1 -> Bus Selector/1
  Bus Selector/1 -> Bus Creator/7  "<Re-InitialisierungsTemp [degC]>"

== system Feuchtesimulation_G21_EU6AGA_rueckgabewerte/NSC/Konfiguration ==
  Bus Creator : BusCreator  Inputs=10
  Bus Creator1 : BusCreator  Inputs=6
  Constant : Constant  Value=A_Kat0
  Constant1 : Constant  Value=l_Kat0
  Constant10 : Constant  Value=Mat_Kat0.lamda
  Constant11 : Constant  Value=beladungskennfeld.maxAdsBel_prz
  Constant12 : Constant  Value=Kat0_Anzahl_Zonen
  Constant13 : Constant  Value=Mat_Kat0.AeffFaktor
  Constant14 : Constant  Value=99
  Constant2 : Constant  Value=Mat_Kat0.beladung
  Constant3 : Constant  Value=-1
  Constant4 : Constant  Value=m_h2o_kat0_kond
  Constant5 : Constant  Value=m_zeolith_kat0_zone
  Constant6 : Constant  Value=m_h2o_kat0_ads
  Constant7 : Constant  Value=m_zKat0
  Constant8 : Constant  Value=Mat_Kat0.c_c
  Constant9 : Constant  Value=Mat_Kat0.c_T
  From Workspace : FromWorkspace  VariableName=T_vCSF
  Terminator : Terminator
  Konfiguration : Outport  VectorParamsAs1DForOutWhenUnconnected=off
  wires:
  Constant10/1 -> Bus Creator1/5  "Wärmeleitfähigkeit [W/mK]"
  Constant13/1 -> Bus Creator1/1  "AeffFaktor [-]"
  Constant7/1 -> Bus Creator/8  "Masse Bauteil pro Zone [kg]"
  Bus Creator1/1 -> Bus Creator/10  "Material Bauteil"
  Constant1/1 -> Bus Creator/2  "Gesamtlänge Bauteil [m]"
  Constant12/1 -> Bus Creator/3  "Anzahl Zonen [-]"
  Bus Creator/1 -> Konfiguration/1
  Constant9/1 -> Bus Creator1/4  "Wärmekapazität KL Temperatur [°C]"
  Constant8/1 -> Bus Creator1/3  "Wärmekapazität Kennlienie [kJ/kgK]"
  Constant2/1 -> Bus Creator1/2  "Max KondBeladung [kg/kg]"
  Constant5/1 -> Bus Creator/6  "Masse Zeolith pro Zone [kg]"
  Constant4/1 -> Bus Creator/5  "Masse Wasser Kondensation start [kg]"
  Constant6/1 -> Bus Creator/7  "Masse Wasser Adsorption start [kg]"
  Constant/1 -> Bus Creator/1  "Querschnittsfläche Bauteil [m2]"
  Constant11/1 -> Bus Creator1/6  "MaxAdsBelGrad [%]"
  Constant3/1 -> Bus Creator/4  "dummy"
  From Workspace/1 -> Bus Creator/9  "Re-InitialisierungsTemp [degC]"
  Constant14/1 -> Terminator/1  "Re-InitialisierungsTemp [degC]"

== system Feuchtesimulation_G21_EU6AGA_rueckgabewerte/NSC/Subsystem ==
  Bel_Ads_% : Inport
  Konfig : Inport  Port=2
  Bus Selector : BusSelector  OutputSignals=Masse Zeolith pro Zone [kg],Material Bauteil.MaxAdsBelGrad [%]
  Gain4 : Gain  Gain=0.1
  Multiply : Product  Inputs=3
  m_H2OAds_g : Outport  VectorParamsAs1DForOutWhenUnconnected=off
  wires:
  Gain4/1 -> m_H2OAds_g/1  "m_Wasser_g"
  Konfig/1 -> Bus Selector/1
  Bel_Ads_%/1 -> Multiply/1
  Bus Selector/2 -> Multiply/3  "<MaxAdsBelGrad [%]>"
  Bus Selector/1 -> Multiply/2  "<Masse Zeolith pro Zone [kg]>"
  Multiply/1 -> Gain4/1  "m*10000_kg"

== system Feuchtesimulation_G21_EU6AGA_rueckgabewerte/NSC/Subsystem1 ==
  Bel_Ads_% : Inport
  Konfig : Inport  Port=2
  Bus Selector : BusSelector  OutputSignals=Masse Zeolith pro Zone [kg],Material Bauteil.MaxAdsBelGrad [%]
  Gain4 : Gain  Gain=0.1
  Multiply : Product  Inputs=3
  m_H2OAds_g : Outport  VectorParamsAs1DForOutWhenUnconnected=off
  wires:
  Gain4/1 -> m_H2OAds_g/1  "m_Wasser_g"
  Konfig/1 -> Bus Selector/1
  Bel_Ads_%/1 -> Multiply/1
  Bus Selector/2 -> Multiply/3  "<MaxAdsBelGrad [%]>"
  Bus Selector/1 -> Multiply/2  "<Masse Zeolith pro Zone [kg]>"
  Multiply/1 -> Gain4/1  "m*10000_kg"

== system Feuchtesimulation_G21_EU6AGA_rueckgabewerte/NSC/kgph to kgps ==
  kgph : Inport
  Constant : Constant  Value=3600
  dm_kgps : Product  Inputs=*/
  kgps : Outport  VectorParamsAs1DForOutWhenUnconnected=off
  wires:
  Constant/1 -> dm_kgps/2
  kgph/1 -> dm_kgps/1
  dm_kgps/1 -> kgps/1

== system Feuchtesimulation_G21_EU6AGA_rueckgabewerte/Relative Feuchte [%]/Limit Sättigungsdampfdruck ==
  note: Hier wird der Maximale Sättigungsdampfdruck limitiert, da sonst in der
      | berechnung eine Singularität auftritt. Ist der Sättigungsdampfdruck gleich
      | dem Druck, ist der maximale Feuchtegehalt erreicht.
  Druck [mbar] : Inport
  Sättigungsdampfdruck [mbar] : Inport  Port=2
  Sum : Sum  Inputs=|+-
  Switch : Switch  Criteria=u2 > Threshold  RndMeth=Simplest  SaturateOnIntegerOverflow=on  InputSameDT=on
  Sättigungsdampfdruck Limitiert [mbar] : Outport  VectorParamsAs1DForOutWhenUnconnected=off
  wires:
  Druck [mbar]/1 -> Switch/3, Sum/1
  Sättigungsdampfdruck [mbar]/1 -> Switch/1, Sum/2
  Sum/1 -> Switch/2
  Switch/1 -> Sättigungsdampfdruck Limitiert [mbar]/1

== system Feuchtesimulation_G21_EU6AGA_rueckgabewerte/Relative Feuchte [%]1/Limit Sättigungsdampfdruck ==
  note: Hier wird der Maximale Sättigungsdampfdruck limitiert, da sonst in der
      | berechnung eine Singularität auftritt. Ist der Sättigungsdampfdruck gleich
      | dem Druck, ist der maximale Feuchtegehalt erreicht.
  Druck [mbar] : Inport
  Sättigungsdampfdruck [mbar] : Inport  Port=2
  Sum : Sum  Inputs=|+-
  Switch : Switch  Criteria=u2 > Threshold  RndMeth=Simplest  SaturateOnIntegerOverflow=on  InputSameDT=on
  Sättigungsdampfdruck Limitiert [mbar] : Outport  VectorParamsAs1DForOutWhenUnconnected=off
  wires:
  Druck [mbar]/1 -> Switch/3, Sum/1
  Sättigungsdampfdruck [mbar]/1 -> Switch/1, Sum/2
  Sum/1 -> Switch/2
  Switch/1 -> Sättigungsdampfdruck Limitiert [mbar]/1

== system Feuchtesimulation_G21_EU6AGA_rueckgabewerte/Relative Feuchte [%]2/Limit Sättigungsdampfdruck ==
  note: Hier wird der Maximale Sättigungsdampfdruck limitiert, da sonst in der
      | berechnung eine Singularität auftritt. Ist der Sättigungsdampfdruck gleich
      | dem Druck, ist der maximale Feuchtegehalt erreicht.
  Druck [mbar] : Inport
  Sättigungsdampfdruck [mbar] : Inport  Port=2
  Sum : Sum  Inputs=|+-
  Switch : Switch  Criteria=u2 > Threshold  RndMeth=Simplest  SaturateOnIntegerOverflow=on  InputSameDT=on
  Sättigungsdampfdruck Limitiert [mbar] : Outport  VectorParamsAs1DForOutWhenUnconnected=off
  wires:
  Druck [mbar]/1 -> Switch/3, Sum/1
  Sättigungsdampfdruck [mbar]/1 -> Switch/1, Sum/2
  Sum/1 -> Switch/2
  Switch/1 -> Sättigungsdampfdruck Limitiert [mbar]/1

== system Feuchtesimulation_G21_EU6AGA_rueckgabewerte/Relative Feuchte [%]3/Limit Sättigungsdampfdruck ==
  note: Hier wird der Maximale Sättigungsdampfdruck limitiert, da sonst in der
      | berechnung eine Singularität auftritt. Ist der Sättigungsdampfdruck gleich
      | dem Druck, ist der maximale Feuchtegehalt erreicht.
  Druck [mbar] : Inport
  Sättigungsdampfdruck [mbar] : Inport  Port=2
  Sum : Sum  Inputs=|+-
  Switch : Switch  Criteria=u2 > Threshold  RndMeth=Simplest  SaturateOnIntegerOverflow=on  InputSameDT=on
  Sättigungsdampfdruck Limitiert [mbar] : Outport  VectorParamsAs1DForOutWhenUnconnected=off
  wires:
  Druck [mbar]/1 -> Switch/3, Sum/1
  Sättigungsdampfdruck [mbar]/1 -> Switch/1, Sum/2
  Sum/1 -> Switch/2
  Switch/1 -> Sättigungsdampfdruck Limitiert [mbar]/1

== system Feuchtesimulation_G21_EU6AGA_rueckgabewerte/Relative Feuchte [%]4/Limit Sättigungsdampfdruck ==
  note: Hier wird der Maximale Sättigungsdampfdruck limitiert, da sonst in der
      | berechnung eine Singularität auftritt. Ist der Sättigungsdampfdruck gleich
      | dem Druck, ist der maximale Feuchtegehalt erreicht.
  Druck [mbar] : Inport
  Sättigungsdampfdruck [mbar] : Inport  Port=2
  Sum : Sum  Inputs=|+-
  Switch : Switch  Criteria=u2 > Threshold  RndMeth=Simplest  SaturateOnIntegerOverflow=on  InputSameDT=on
  Sättigungsdampfdruck Limitiert [mbar] : Outport  VectorParamsAs1DForOutWhenUnconnected=off
  wires:
  Druck [mbar]/1 -> Switch/3, Sum/1
  Sättigungsdampfdruck [mbar]/1 -> Switch/1, Sum/2
  Sum/1 -> Switch/2
  Switch/1 -> Sättigungsdampfdruck Limitiert [mbar]/1

== system Feuchtesimulation_G21_EU6AGA_rueckgabewerte/Relative Feuchte [%]5/Limit Sättigungsdampfdruck ==
  note: Hier wird der Maximale Sättigungsdampfdruck limitiert, da sonst in der
      | berechnung eine Singularität auftritt. Ist der Sättigungsdampfdruck gleich
      | dem Druck, ist der maximale Feuchtegehalt erreicht.
  Druck [mbar] : Inport
  Sättigungsdampfdruck [mbar] : Inport  Port=2
  Sum : Sum  Inputs=|+-
  Switch : Switch  Criteria=u2 > Threshold  RndMeth=Simplest  SaturateOnIntegerOverflow=on  InputSameDT=on
  Sättigungsdampfdruck Limitiert [mbar] : Outport  VectorParamsAs1DForOutWhenUnconnected=off
  wires:
  Druck [mbar]/1 -> Switch/3, Sum/1
  Sättigungsdampfdruck [mbar]/1 -> Switch/1, Sum/2
  Sum/1 -> Switch/2
  Switch/1 -> Sättigungsdampfdruck Limitiert [mbar]/1

== system Feuchtesimulation_G21_EU6AGA_rueckgabewerte/Relative Feuchte [%]6/Limit Sättigungsdampfdruck ==
  note: Hier wird der Maximale Sättigungsdampfdruck limitiert, da sonst in der
      | berechnung eine Singularität auftritt. Ist der Sättigungsdampfdruck gleich
      | dem Druck, ist der maximale Feuchtegehalt erreicht.
  Druck [mbar] : Inport
  Sättigungsdampfdruck [mbar] : Inport  Port=2
  Sum : Sum  Inputs=|+-
  Switch : Switch  Criteria=u2 > Threshold  RndMeth=Simplest  SaturateOnIntegerOverflow=on  InputSameDT=on
  Sättigungsdampfdruck Limitiert [mbar] : Outport  VectorParamsAs1DForOutWhenUnconnected=off
  wires:
  Druck [mbar]/1 -> Switch/3, Sum/1
  Sättigungsdampfdruck [mbar]/1 -> Switch/1, Sum/2
  Sum/1 -> Switch/2
  Switch/1 -> Sättigungsdampfdruck Limitiert [mbar]/1

== system Feuchtesimulation_G21_EU6AGA_rueckgabewerte/Rohr nach SCR/Konfiguration2 ==
  Bus Creator : BusCreator  Inputs=13
  Constant : Constant  Value=Rohr2.Mantelflaeche_innen
  Constant1 : Constant  Value=Rohr2.Mantelflaeche_aussen
  Constant10 : Constant  Value=99
  Constant12 : Constant  Value=Rohr2.Laenge_Abschnitt
  Constant15 : Constant  Value=Rohr2.Waermeleitquerschnitt
  Constant2 : Constant  Value=Rohr2.StroemungsdurchmesserEff
  Constant3 : Constant  Value=Rohr2.thermWidIso
  Constant4 : Constant  Value=Rohr2.Masse_Wasser_start
  Constant5 : Constant  Value=Rohr2.LambdaRohr
  Constant6 : Constant  Value=Rohr2.MasseRohr
  Constant7 : Constant  Value=0
  Constant8 : Constant  Value=Rohr2.Waermekapazitaet
  Constant9 : Constant  Value=Rohr2.thermWidRohr
  From Workspace1 : FromWorkspace  VariableName=T_nSCR
  Terminator : Terminator
  Konfiguration : Outport  VectorParamsAs1DForOutWhenUnconnected=off
  wires:
  Bus Creator/1 -> Konfiguration/1
  Constant/1 -> Bus Creator/1  "Mantelfläche innen [m2]"
  Constant1/1 -> Bus Creator/2  "Mantelfläche außen [m2]"
  Constant4/1 -> Bus Creator/5  "Masse Wasser start [kg]"
  Constant12/1 -> Bus Creator/3  "Länge RohrSegment [m]"
  Constant15/1 -> Bus Creator/11  "Wärmeleitquerschnitt Rohr [m2]"
  Constant2/1 -> Bus Creator/7  "gleichwertiger Strömungsdurchmesser [m]"
  Constant5/1 -> Bus Creator/8  "Wärmeleitfähigkeit [W/mK]"
  Constant6/1 -> Bus Creator/9  "Masse Rohr [kg]"
  Constant8/1 -> Bus Creator/10  "Wärmekapazität Rohr [J/kgK]"
  From Workspace1/1 -> Bus Creator/13  "Re-InitialisierungsTemp [degC]"
  Constant3/1 -> Bus Creator/4  "r_thermWidIso_m2K/W"
  Constant9/1 -> Bus Creator/6  "r_thermWidRohr_m2K/W"
  Constant7/1 -> Bus Creator/12  "dummy"
  Constant10/1 -> Terminator/1  "Re-InitialisierungsTemp [degC]"
